simulink model "filterdesign"  (R2025b)
settings: Solver=VariableStepAuto  StartTime=0.0  StopTime=5  FixedStep=4.878e-7  RelTol=1e-3
undefined symbols (not defined in the file): dspblkCoreblockFVToolHelper, gcbh
settings Model: Creator=ashaydwivedi  LastModifiedBy=ashaydwivedi

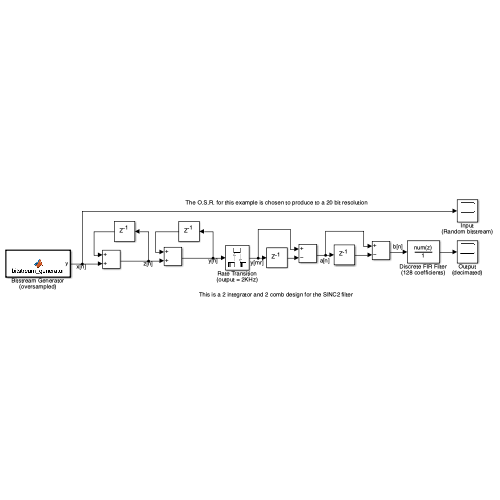
[thumbnail: Simulink's stored preview of the top-level diagram]
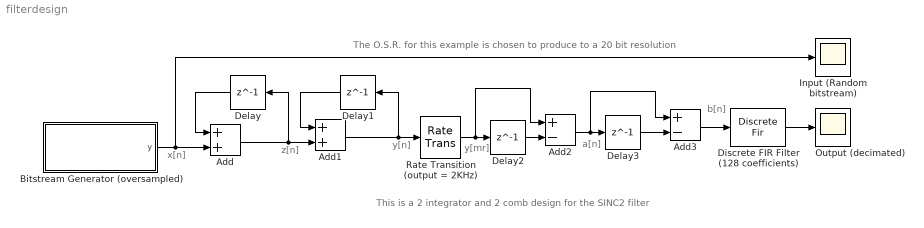
== system filterdesign ==
  note: x[n]
  note: The O.S.R. for this example is chosen to produce to a 20 bit resolution
  note: This is a 2 integrator and 2 comb design for the SINC2 filter
  note: z[n]
  note: y[n]
  note: y[mr]
  note: a[n]
  note: b[n]
  Add : Sum
  Add1 : Sum
  Add2 : Sum  Inputs=+-
  Add3 : Sum  Inputs=+-
  Bitstream Generator (oversampled) : MATLAB Function  TreatAsAtomicUnit=on  SystemSampleTime=4.8780487804878046e-7
  Delay{,1..3} (4 alike) : Delay  DelayLength=1  InitialCondition=0
  Discrete FIR Filter (128 coefficients) : DiscreteFir  LoadFcn=dspblkCoreblockFVToolHelper(gcbh,'load');  Coefficients=[0.0078125 0.0078125 0.0078125 0.0078125 0.0078125 0.0078125 0.0078125 0.0078125 0.0078125 0.0078125 0.0078125 0.0078125 0.0078125 0.0078125 0.0078125 0.0078125 0.0078125 0.0078125 0.0078125 0.0078125 0.0078125 0.0078125 0.0078125 0.0078125 0.0078125 0.0078125 0.0078125 0.0078125 0.0078125 0.0078125 0.0078125 0.0078125 0.0078125 0.0078125 0.0078125 0.0078125 0.0078125 0.0078125 0.0078125 0.0078125 0.0078125 0.0078125 0.0078125 0.0078125 0.0078125 0.0078125 0.0078125 0.0078125 0.0078125 0.0078125 0.0078125 0.0078125 0.0078125 0.0078125 0.0078125 0.0078125 0.0078125 0.0078125 0.0078125 0.0078125 0.0078125 0.0078125 0.0078125 0.0078125 0.0078125 0.0078125 0.0078125 0.0078125 0.0078125 0.0078125 0.0078125 0.0078125 0.0078125 0.0078125 0.0078125 0.0078125 0.0078125 0.0078125 0.0078125 0.0078125 0.0078125 0.0078125 0.0078125 0.0078125 0.0078125 0.0078125 0.0078125 0.0078125 0.0078125 0.0078125 0.0078125 0.0078125 0.0078125 0.0078125 0.0078125 0.0078125 0.0078125 0.0078125 0.0078125 0.0078125 0.0078125 0.0078125 0.0078125 0.0078125 0.0078125 0.0078125 0.0078125 0.0078125 0.0078125 0.0078125 0.0078125 0.0078125 0.0078125 0.0078125 0.0078125 0.0078125 0.0078125 0.0078125 0.0078125 0.0078125 0.0078125 0.0078125 0.0078125 0.0078125 0.0078125 0.0078125 0.0078125 0.0078125 0.0078125 0.0078125 0.0078125 0.0078125 0.0078125 0.0078125 0.0078125 0.0078125]
      settings: CopyFcn=dspblkCoreblockFVToolHelper(gcbh,'copy');  DeleteFcn=dspblkCoreblockFVToolHelper(gcbh,'close');  ModelCloseFcn=dspblkCoreblockFVToolHelper(gcbh,'close');  PreSaveFcn=dspblkCoreblockFVToolHelper(gcbh,'presave');  PostSaveFcn=dspblkCoreblockFVToolHelper(gcbh,'postsave');  CloseFcn=dspblkCoreblockFVToolHelper(gcbh,'close');
  Input (Random bitstream) : Scope
      settings: ActiveDisplayYMinimum=-1.25  ActiveDisplayYMaximum=1.25
  Output (decimated) : Scope
      settings: ActiveDisplayYMinimum=-44183.3515625  ActiveDisplayYMaximum=33746.2578125
  Rate Transition (output = 2KHz) : RateTransition  OutPortSampleTime=1/2000
  wires:
  Discrete FIR Filter (128 coefficients)/1 -> Output (decimated)/1
  Add1/1 -> Delay1/1, Rate Transition (output = 2KHz)/1
  Delay/1 -> Add/1
  Bitstream Generator (oversampled)/1(y) -> Add/2, Input (Random bitstream)/1
  Add/1 -> Add1/2, Delay/1
  Delay1/1 -> Add1/1
  Rate Transition (output = 2KHz)/1 -> Delay2/1, Add2/1
  Delay2/1 -> Add2/2
  Add2/1 -> Add3/1, Delay3/1
  Delay3/1 -> Add3/2
  Add3/1 -> Discrete FIR Filter (128 coefficients)/1

== matlab function filterdesign/Bitstream Generator (oversampled) ==
  data: y output
function y = bitstream_generator()
% High entropy ±1 bitstream

persistent s1 s2
if isempty(s1)
    s1 = 0;
end
if isempty(s2)
    s2 = 0;
end

% Full strength White Noise
w = randn();          

% Two fast internal states
s1 = 0.8 * s1 + w;    
s2 = 0.6 * s2 + s1 + 0.2*w;

% Final excitation
v = 0.5*s2 + 0.3*w + 0.2*randn();

% Quantizer to generate the bits
if v >= 0
    y = 1;
else
    y = -1;
end
